simulink model "ME19B085_project_2"  (R2021a)
settings: Solver=VariableStepAuto  StartTime=0.0  StopTime=10.0  RelTol=1e-3
settings Model: Creator=Ashwin Dev  LastModifiedBy=Ashwin Dev
settings SolverCC: ZeroCrossAlgorithm=Adaptive
settings DebuggingCC: IgnoredZcDiagnostic=none

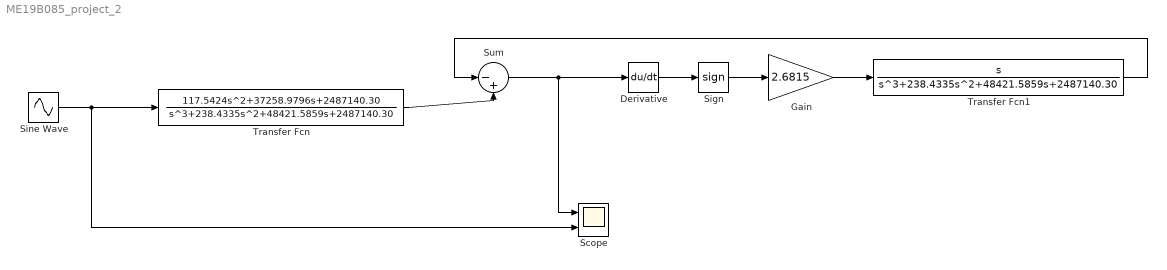
== system ME19B085_project_2 ==
  Derivative : Derivative
  Gain : Gain  Gain=2.6815
  Scope : Scope  NumInputPorts=2
  Sign : Signum
  Sine Wave : Sin  SampleTime=0
  Sum : Sum  Inputs=|-+
  Transfer Fcn : TransferFcn  Numerator=[117.5424 37258.9796 2487140.30]  Denominator=[1 238.4335 48421.5859 2487140.30]
  Transfer Fcn1 : TransferFcn  Numerator=[1 0]  Denominator=[1 238.4335 48421.5859 2487140.30]
  wires:
  Sine Wave/1 -> Scope/2, Transfer Fcn/1
  Transfer Fcn/1 -> Sum/2
  Sum/1 -> Scope/1, Derivative/1
  Derivative/1 -> Sign/1
  Sign/1 -> Gain/1
  Gain/1 -> Transfer Fcn1/1
  Transfer Fcn1/1 -> Sum/1
